simulink model "ReadWriteSerial"  (R2022b)
settings: Solver=FixedStepAuto  StartTime=0.0  StopTime=inf  FixedStep=0.01  RelTol=1e-3
undefined symbols (not defined in the file): CR, LF
libraries: instrumentseriallib x3
settings Model: ExtModeTrigDuration=2  Creator=mario  LastModifiedBy=mario
settings OptimizationCC: EnhancedBackFolding=on  PassReuseOutputArgsAs=Individual arguments  ZeroExternalMemoryAtStartup=off  ZeroInternalMemoryAtStartup=off  MaxStackSize=64  OptimizeBlockOrder=speed  DifferentSizesBufferReuse=on  OptimizationCustomize=off  EfficientTunableParamExpr=on
settings DebuggingCC: ParameterTunabilityLossMsg=error
settings HardwareCC: ProdBitPerPointer=32  ProdBitPerSizeT=32  ProdBitPerPtrDiffT=32  ProdLargestAtomicInteger=Long  ProdLargestAtomicFloat=Double  ProdWordSize=32  ProdHWDeviceType=ARM Compatible->ARM Cortex  UseEmbeddedCoderFeatures=off
settings SFSimCC: MATLABDynamicMemAlloc=off
settings RTWCC: Description=Embedded Coder  SystemTargetFile=ert.tlc  HardwareBoard=Arduino Due  TLCOptions=-aInlineSetEventsForThisBaseRateFcn=TLC_FALSE -aSuppressMultiTaskScheduler=TLC_FALSE -aRateBasedStepFcn=1  TemplateMakefile=ert_default_tmf  Toolchain=Arduino ARM
settings CodeAppCC: ForceParamTrailComments=on  IgnoreCustomStorageClasses=off  OperatorAnnotations=on  SimulinkDataObjDesc=on  SFDataObjDesc=on  InsertBlockDesc=on
settings ERTTargetCC: SupportContinuousTime=on  SupportNonInlinedSFcns=on  SupportVariableSizeSignals=on  ExtModeTransport=3  ExtModeStaticAlloc=on  ExtModeAutomaticAllocSize=off  ExtModeStaticAllocSize=24576  ExtModeMexFile=ext_xcp  ExtModeIntrfLevel=Level2 - Open

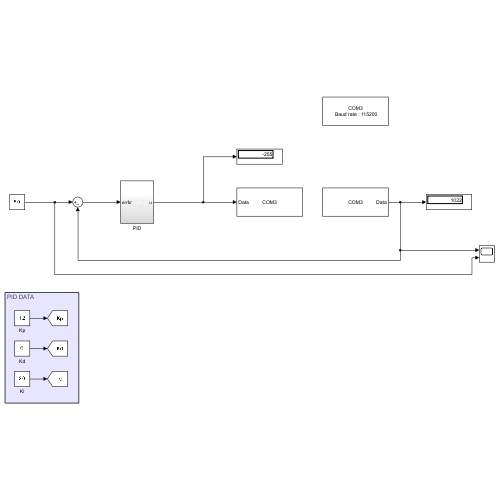
[thumbnail: Simulink's stored preview of the top-level diagram]
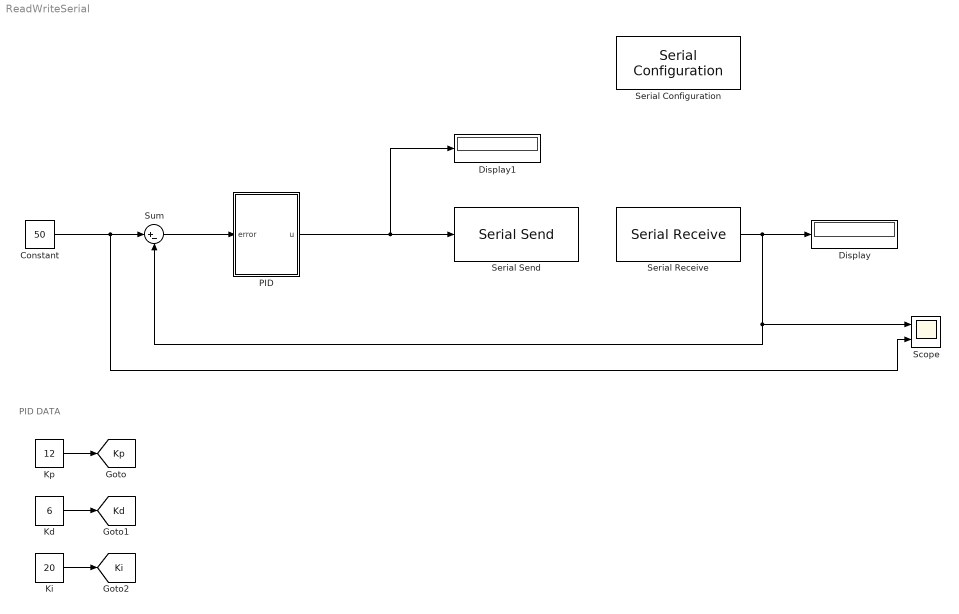
== system ReadWriteSerial ==
  note: PID DATA
  Constant : Constant  Value=50  OutDataTypeStr=single
  Display : Display
  Display1 : Display
  Kd : Constant  Value=6
  Ki : Constant  Value=20
  Kp : Constant  Value=12
  PID : Subsystem
  Scope : Scope  NumInputPorts=2
  Serial Configuration : instrumentseriallib/Serial Configuration  Priority=-200000  PortSel=COM3  Port=COM3  ComPort=COM3  BaudRate=115200  DataBits=8  Parity=none  StopBits=1  ByteOrder=little-endian  FlowControl=none  Timeout=10  SimulateUsing=Interpreted execution  BlockInModel=on  aMode=1
  Serial Receive : instrumentseriallib/Serial Receive  Priority=1  PortSel=COM3  Port=COM3  ComPort=COM3  DataType=single  SaveDataType=uint8  ToggleHeader=off  Header='R'  ToggleTerminator=on  Terminator=CR/LF ('\r\n')  CustomTerminator=[]  InputFormat=Row major  ToggleDataSize=on  DataSize=[1 1]  EnableBlockingMode=on  ActionDataUnavailable=Output last received value  ActionWhenDataUnavailable=Output last received value  CustomValue=0  SampleTime=0.01  SimulateUsing=Interpreted execution  BlockInModel=on  aMode=1
  Serial Send : instrumentseriallib/Serial Send  Priority=1  PortSel=COM3  Port=COM3  ComPort=COM3  Header=[]  Terminator=LF ('\n')  CustomTerminator=[]  EnableBlockingMode=on  SimulateUsing=Interpreted execution  BlockInModel=on  aMode=1
  Sum : Sum  Inputs=|+-
  tag scope: Kd=global, Ki=global, Kp=global
  wires:
  Serial Receive/1 -> Display/1, Scope/1, Sum/2
  Constant/1 -> Scope/2, Sum/1
  Kp/1 -> [Kp]
  Ki/1 -> [Ki]
  Kd/1 -> [Kd]
  Sum/1 -> PID/1(error)
  PID/1(u) -> Display1/1, Serial Send/1

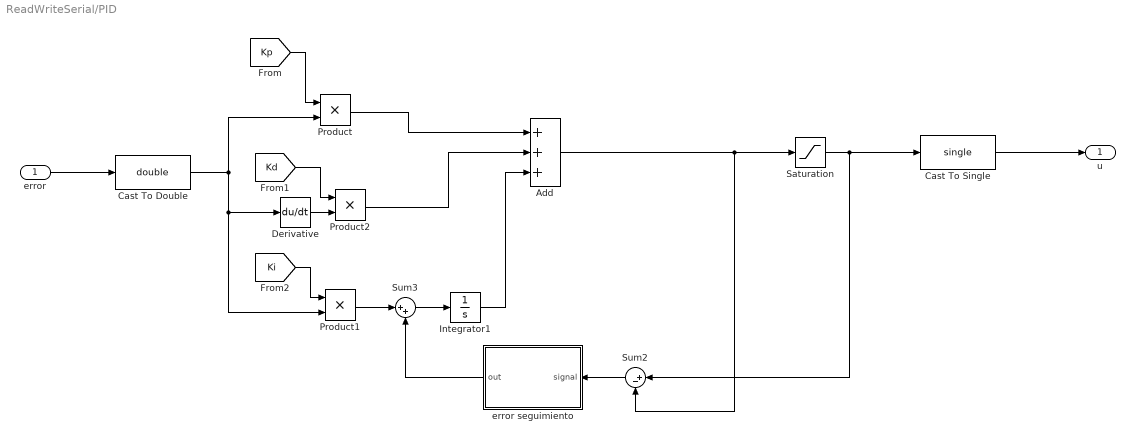
== system ReadWriteSerial/PID ==
  error : Inport
  Add : Sum  Inputs=+++
  Cast To Double : DataTypeConversion  OutDataTypeStr=double  SaturateOnIntegerOverflow=off  RndMeth=Floor
  Cast To Single : DataTypeConversion  OutDataTypeStr=single  SaturateOnIntegerOverflow=off  RndMeth=Floor
  Derivative : Derivative
  Integrator1 : Integrator
  Product : Product
  Product1 : Product
  Product2 : Product
  Saturation : Saturate  UpperLimit=255  LowerLimit=-255
  Sum2 : Sum  Inputs=|+-
  Sum3 : Sum  Inputs=|++
  error seguimiento : Subsystem
  u : Outport
  wires:
  error/1 -> Cast To Double/1
  [Kp] -> Product/1
  [Kd] -> Product2/1
  Product/1 -> Add/1
  [Ki] -> Product1/1
  Cast To Double/1 -> Product/2, Product1/2, Derivative/1
  Derivative/1 -> Product2/2
  Saturation/1 -> Cast To Single/1, Sum2/1
  Product1/1 -> Sum3/1
  Sum3/1 -> Integrator1/1
  Add/1 -> Saturation/1, Sum2/2
  Sum2/1 -> error seguimiento/1(signal)
  Cast To Single/1 -> u/1
  error seguimiento/1(out) -> Sum3/2
  Product2/1 -> Add/2
  Integrator1/1 -> Add/3

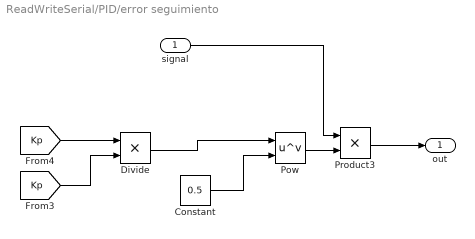
== system ReadWriteSerial/PID/error seguimiento ==
  signal : Inport
  Constant : Constant  Value=0.5
  Divide : Product  Inputs=**
  Pow : Math  Operator=pow  SignedPower=on  RndMeth=Zero
  Product3 : Product
  out : Outport
  wires:
  Divide/1 -> Pow/1
  Product3/1 -> out/1
  Pow/1 -> Product3/2
  [Kp] -> Divide/2
  signal/1 -> Product3/1
  [Kp] -> Divide/1
  Constant/1 -> Pow/2
